simulink model "foc_prescribed_v2"  (R2015a)
settings: Solver=ode23tb  StartTime=0  StopTime=4  MaxStep=0.0001  RelTol=1e-06  AbsTol=1e-08
settings Model: Creator=user  LastModifiedBy=user
settings DataIOCC: SaveOutput=off  SaveTime=off

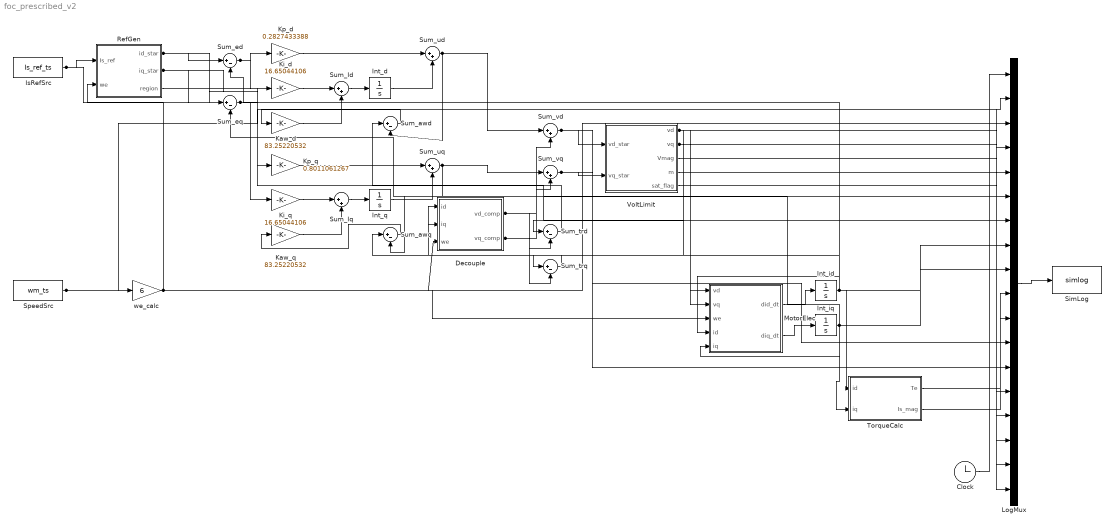
== system foc_prescribed_v2 ==
  Clock : Clock
  Decouple : MATLAB Function  TreatAsAtomicUnit=on
  Int_d : Integrator
  Int_id : Integrator
  Int_iq : Integrator
  Int_q : Integrator
  IsRefSrc : FromWorkspace  VariableName=Is_ref_ts  SampleTime=0  OutputAfterFinalValue=Holding final value
  Kaw_d : Gain  Gain=83.25220532
  Kaw_q : Gain  Gain=83.25220532
  Ki_d : Gain  Gain=16.65044106
  Ki_q : Gain  Gain=16.65044106
  Kp_d : Gain  Gain=0.2827433388
  Kp_q : Gain  Gain=0.8011061267
  LogMux : Mux  Inputs=18
  MotorElec : MATLAB Function  TreatAsAtomicUnit=on
  RefGen : MATLAB Function  TreatAsAtomicUnit=on
  SimLog : ToWorkspace  VariableName=simlog  SampleTime=-1
  SpeedSrc : FromWorkspace  VariableName=wm_ts  SampleTime=0  OutputAfterFinalValue=Holding final value
  Sum_Id : Sum  Inputs=|++
  Sum_Iq : Sum  Inputs=|++
  Sum_awd : Sum  Inputs=|+-
  Sum_awq : Sum  Inputs=|+-
  Sum_ed : Sum  Inputs=|+-
  Sum_eq : Sum  Inputs=|+-
  Sum_trd : Sum  Inputs=|+-
  Sum_trq : Sum  Inputs=|+-
  Sum_ud : Sum  Inputs=|++
  Sum_uq : Sum  Inputs=|++
  Sum_vd : Sum  Inputs=|++
  Sum_vq : Sum  Inputs=|++
  TorqueCalc : MATLAB Function  TreatAsAtomicUnit=on
  VoltLimit : MATLAB Function  TreatAsAtomicUnit=on
  we_calc : Gain  Gain=6
  wires:
  SpeedSrc/1 -> we_calc/1, LogMux/2
  IsRefSrc/1 -> RefGen/1(Is_ref), LogMux/4
  we_calc/1 -> RefGen/2(we), Decouple/3(we), MotorElec/3(we), LogMux/3
  RefGen/1(id_star) -> Sum_ed/1, LogMux/5
  Int_id/1 -> Sum_ed/2, Decouple/1(id), MotorElec/4(id), TorqueCalc/1(id), LogMux/8
  RefGen/2(iq_star) -> Sum_eq/1, LogMux/6
  Int_iq/1 -> Sum_eq/2, Decouple/2(iq), MotorElec/5(iq), TorqueCalc/2(iq), LogMux/9
  Sum_ed/1 -> Kp_d/1, Ki_d/1
  Kp_d/1 -> Sum_ud/1
  Int_d/1 -> Sum_ud/2
  Ki_d/1 -> Sum_Id/1
  Kaw_d/1 -> Sum_Id/2
  Sum_Id/1 -> Int_d/1
  Sum_trd/1 -> Sum_awd/1
  Sum_ud/1 -> Sum_awd/2, Sum_vd/1
  Sum_awd/1 -> Kaw_d/1
  Sum_eq/1 -> Kp_q/1, Ki_q/1
  Kp_q/1 -> Sum_uq/1
  Int_q/1 -> Sum_uq/2
  Ki_q/1 -> Sum_Iq/1
  Kaw_q/1 -> Sum_Iq/2
  Sum_Iq/1 -> Int_q/1
  Sum_trq/1 -> Sum_awq/1
  Sum_uq/1 -> Sum_awq/2, Sum_vq/1
  Sum_awq/1 -> Kaw_q/1
  Decouple/1(vd_comp) -> Sum_vd/2, Sum_trd/2
  Decouple/2(vq_comp) -> Sum_vq/2, Sum_trq/2
  Sum_vd/1 -> VoltLimit/1(vd_star), LogMux/12
  Sum_vq/1 -> VoltLimit/2(vq_star), LogMux/13
  VoltLimit/1(vd) -> Sum_trd/1, MotorElec/1(vd), LogMux/14
  VoltLimit/2(vq) -> Sum_trq/1, MotorElec/2(vq), LogMux/15
  MotorElec/1(did_dt) -> Int_id/1
  MotorElec/2(diq_dt) -> Int_iq/1
  Clock/1 -> LogMux/1
  RefGen/3(region) -> LogMux/7
  TorqueCalc/2(Is_mag) -> LogMux/10
  TorqueCalc/1(Te) -> LogMux/11
  VoltLimit/3(Vmag) -> LogMux/16
  VoltLimit/4(m) -> LogMux/17
  VoltLimit/5(sat_flag) -> LogMux/18
  LogMux/1 -> SimLog/1

== matlab function foc_prescribed_v2/Decouple ==
  data: id input; vd_comp output; iq input; we input; vq_comp output
function [vd_comp, vq_comp] = Decouple(id, iq, we)
%#codegen
% Feed-forward cancellation of the speed-dependent cross-coupling terms
%   vd = Rs*id + Ld*did/dt - we*Lq*iq
%   vq = Rs*iq + Lq*diq/dt + we*(Ld*id + lam)
% so that each axis presents a first-order plant to its PI controller.
vd_comp = -we*0.000255*iq;
vq_comp =  we*(9e-05*id + 0.0385);
end

== matlab function foc_prescribed_v2/RefGen ==
  data: Is_ref input; id_star output; we input; iq_star output; region output
function [id_star, iq_star, region] = RefGen(Is_ref, we)
%#codegen
% Single authoritative source of the current references.
% Delegates to the validated IPMSM_REF_GEN; machine parameters are
% injected by BUILD_FOC_MODEL from IPMSM_PARAMS.
[id_star, iq_star, region] = ipmsm_ref_gen(Is_ref, we, 0.0053, 9e-05, 0.000255, 0.0385, 207.8460969, 430, 1);
end

== matlab function foc_prescribed_v2/VoltLimit ==
  data: vd_star input; vd output; vq_star input; vq output; Vmag output; m output; sat_flag output
function [vd, vq, Vmag, m, sat_flag] = VoltLimit(vd_star, vq_star)
%#codegen
% SVPWM linear-range limit, applied in dq. The inverse Park transform is
% a rotation, so |[valpha;vbeta]| = |[vd;vq]| and clipping here is
% identical to clipping in the stationary frame.
% The direction of the voltage vector is preserved (magnitude scaling),
% which is the standard minimum-distortion choice.
Vmax = 207.8460969;
Vmag = sqrt(vd_star^2 + vq_star^2);
m    = Vmag/Vmax;
if Vmag <= Vmax
    vd = vd_star; vq = vq_star; sat_flag = 0;
else
    s = Vmax/Vmag; vd = vd_star*s; vq = vq_star*s; sat_flag = 1;
end
end

== matlab function foc_prescribed_v2/MotorElec ==
  data: vd input; did_dt output; vq input; we input; id input; iq input; diq_dt output
function [did_dt, diq_dt] = MotorElec(vd, vq, we, id, iq)
%#codegen
% IPMSM dq electrical dynamics (magnetically linear).
did_dt = (vd - 0.0053*id + we*0.000255*iq) / 9e-05;
diq_dt = (vq - 0.0053*iq - we*(9e-05*id + 0.0385)) / 0.000255;
end

== matlab function foc_prescribed_v2/TorqueCalc ==
  data: id input; Te output; iq input; Is_mag output
function [Te, Is_mag] = TorqueCalc(id, iq)
%#codegen
% Te = 1.5*p*[ lam*iq + (Ld-Lq)*id*iq ]   (PM term + reluctance term)
Te     = 1.5*6*(0.0385*iq + (9e-05 - 0.000255)*id*iq);
Is_mag = sqrt(id^2 + iq^2);
end
